simulink model "DAC_SIM_LTE"  (R2013b)
settings: Solver=FixedStepDiscrete  SolverMode=SingleTasking  StartTime=0.0  StopTime=N/Fs  RelTol=1e-3
values from neighbouring files (symbols this model uses):
  Tpass = 1/Fpass    (= 3.25520833333e-08)    [Model.m]
undefined symbols (not defined in the file or in its folder): a1, a2, a3, a4, b1, b2, b3, b4, g1, g2, g3, g4
libraries: xbsIndex_r4 x85, dspmlti4 x3, dspsigops x2, simulink x1
(part 1 of 2)
settings Model: Creator=o_cotte  LastModifiedBy=o_cotte

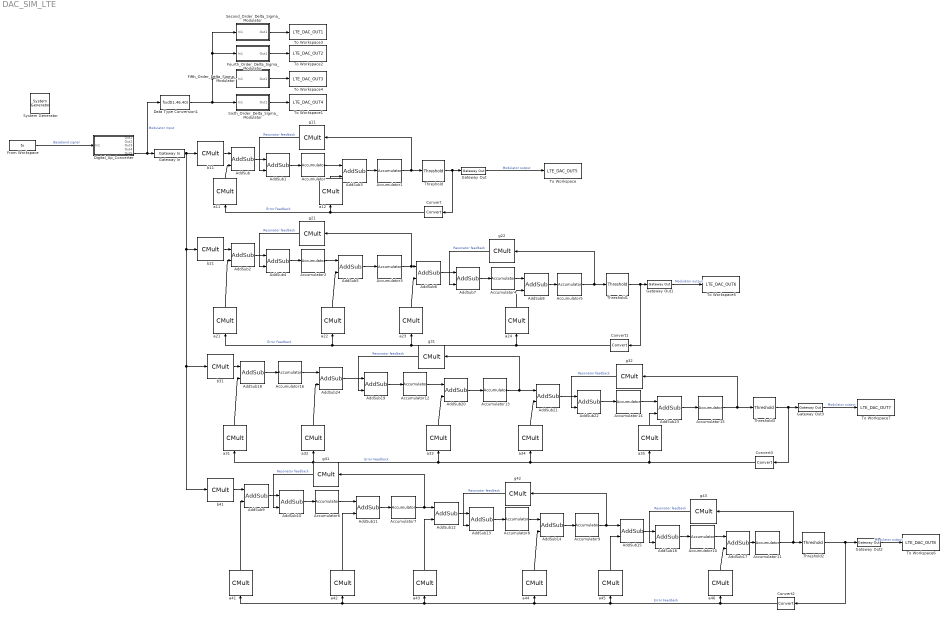
== system DAC_SIM_LTE ==
  " System Generator" : xbsIndex_r4/ System Generator  Tag=genX  xilinxfamily=spartan6  part=xc6slx45  speed=-3  package=csg324  synthesis_tool=XST  clock_wrapper=Clock Enables  directory=./netlist  proj_type=Project Navigator  Synth_file=XST Defaults  Impl_file=ISE Defaults  testbench=off  simulink_period=1/491.52e6  sysclk_period=2.0345052083333335  dcm_input_clock_period=10  incr_netlist=off  trim_vbits=Everywhere in SubSystem  dbl_ovrd=According to Block Masks  core_generation=According to Block Masks  run_coregen=off  deprecated_control=off  eval_field=0  block_type=sysgen
  Accumulator{,1..5,12..16} (11 alike) : xbsIndex_r4/Accumulator  operation=Add  n_bits=46  overflow=Wrap  scale=1  rst=off  infoeditControl=reset for floating point data type must be asserted for a minimum of 2 cycles  hasbypass=off  en=off  latency=0  dbl_ovrd=off  msb_inp=100  msb=100  lsb=-100  use_behavioral_HDL=on  implementation=DSP48  block_type=accum
  Accumulator{6..11} (6 alike) : xbsIndex_r4/Accumulator  operation=Add  n_bits=46  overflow=Wrap  scale=1  rst=off  infoeditControl=reset for floating point data type must be asserted for a minimum of 2 cycles  hasbypass=off  en=off  latency=0  dbl_ovrd=off  msb_inp=100  msb=100  lsb=-100  use_behavioral_HDL=off  implementation=DSP48  block_type=accum
  AddSub{,1..24} (25 alike) : xbsIndex_r4/AddSub  mode=Subtraction  use_carryin=off  use_carryout=off  en=off  latency=0  precision=User Defined  arith_type="Signed  (2's comp)"  n_bits=46  bin_pt=40  quantization=Truncate  overflow=Wrap  dbl_ovrd=off  use_behavioral_HDL=off  hw_selection=DSP48  pipelined=on  block_type=addsub
  Convert{,1..3} (4 alike) : xbsIndex_r4/Convert  gui_display_data_type=Fixed-point  arith_type="Signed  (2's comp)"  n_bits=46  bin_pt=40  float_type=Single  exp_bits=8  fraction_bits=24  quantization=Truncate  overflow=Wrap  en=off  latency=0  dbl_ovrd=off  pipeline=on  block_type=convert
  Data Type Conversion1 : DataTypeConversion  OutDataTypeStr=fixdt(1,46,40)  LockScale=on
  Digital_Up_Converter : Subsystem
  Fifth_Order_Delta_Sigma_Modulator : Subsystem
  Fourth_Order_Delta_Sigma_Modulator : Subsystem
  From Workspace : FromWorkspace  VariableName=tx  SampleTime=Tpass  Interpolate=off  OutputAfterFinalValue=Cyclic repetition
  Gateway In : xbsIndex_r4/Gateway In  gui_display_data_type=Fixed-point  arith_type="Signed  (2's comp)"  n_bits=46  bin_pt=40  preci_type=Single  exp_width=8  frac_width=24  quantization=Truncate  overflow=Saturate  period=1/491.52e6  dbl_ovrd=off  timing_constraint=Data Rate  locs_specified=off  LOCs={}  UseAsADC=off  ADCChannel='1'  inherit_from_input=off  hdl_port=on  block_type=gatewayin
  Gateway Out{,1..3} (4 alike) : xbsIndex_r4/Gateway Out  inherit_from_input=off  hdl_port=on  timing_constraint="Data Rate;  Set 'FAST' Attribute"  locs_specified=off  LOCs={}  UseAsDAC=off  DACChannel='1'  block_type=gatewayout
  Second_Order_Delta_Sigma_Modulator : Subsystem
  Sixth_Order_Delta_Sigma_Modulator : Subsystem
  Threshold{,1..3} (4 alike) : xbsIndex_r4/Threshold  en=off  latency=0  dbl_ovrd=off  block_type=sgn
      settings: infoedit="Presents -1 as output if input is negative; otherwise presents 1.  Output is a two bit signed number."
  To Workspace : ToWorkspace  VariableName=LTE_DAC_OUT5  SampleTime=-1
  To Workspace1 : ToWorkspace  VariableName=LTE_DAC_OUT4  SampleTime=-1
  To Workspace2 : ToWorkspace  VariableName=LTE_DAC_OUT2  SampleTime=-1
  To Workspace3 : ToWorkspace  VariableName=LTE_DAC_OUT1  SampleTime=-1
  To Workspace4 : ToWorkspace  VariableName=LTE_DAC_OUT3  SampleTime=-1
  To Workspace5 : ToWorkspace  VariableName=LTE_DAC_OUT6  SampleTime=-1
  To Workspace6 : ToWorkspace  VariableName=LTE_DAC_OUT8  SampleTime=-1
  To Workspace7 : ToWorkspace  VariableName=LTE_DAC_OUT7  SampleTime=-1
  a11 : xbsIndex_r4/CMult  const=a1(1)  gui_display_data_type=Fixed-point  const_n_bits=46  const_bin_pt=40  float_type=Single  exp_bits=8  fraction_bits=24  en=off  latency=0  precision=User Defined  arith_type="Signed  (2's comp)"  n_bits=46  bin_pt=40  quantization=Truncate  overflow=Wrap  dbl_ovrd=off  use_behavioral_HDL=on  mem_type=Block RAM  pipeline=off  block_type=cmult
  a12 : xbsIndex_r4/CMult  const=a1(2)  gui_display_data_type=Fixed-point  const_n_bits=46  const_bin_pt=40  float_type=Single  exp_bits=8  fraction_bits=24  en=off  latency=0  precision=User Defined  arith_type="Signed  (2's comp)"  n_bits=46  bin_pt=40  quantization=Truncate  overflow=Wrap  dbl_ovrd=off  use_behavioral_HDL=on  mem_type=Block RAM  pipeline=off  block_type=cmult
  a21 : xbsIndex_r4/CMult  const=a2(1)  gui_display_data_type=Fixed-point  const_n_bits=46  const_bin_pt=40  float_type=Single  exp_bits=8  fraction_bits=24  en=off  latency=0  precision=User Defined  arith_type="Signed  (2's comp)"  n_bits=46  bin_pt=40  quantization=Truncate  overflow=Wrap  dbl_ovrd=off  use_behavioral_HDL=on  mem_type=Block RAM  pipeline=off  block_type=cmult
  a22 : xbsIndex_r4/CMult  const=a2(2)  gui_display_data_type=Fixed-point  const_n_bits=46  const_bin_pt=40  float_type=Single  exp_bits=8  fraction_bits=24  en=off  latency=0  precision=User Defined  arith_type="Signed  (2's comp)"  n_bits=46  bin_pt=40  quantization=Truncate  overflow=Wrap  dbl_ovrd=off  use_behavioral_HDL=on  mem_type=Block RAM  pipeline=off  block_type=cmult
  a23 : xbsIndex_r4/CMult  const=a2(3)  gui_display_data_type=Fixed-point  const_n_bits=46  const_bin_pt=40  float_type=Single  exp_bits=8  fraction_bits=24  en=off  latency=0  precision=User Defined  arith_type="Signed  (2's comp)"  n_bits=46  bin_pt=40  quantization=Truncate  overflow=Wrap  dbl_ovrd=off  use_behavioral_HDL=on  mem_type=Block RAM  pipeline=off  block_type=cmult
  a24 : xbsIndex_r4/CMult  const=a2(4)  gui_display_data_type=Fixed-point  const_n_bits=46  const_bin_pt=40  float_type=Single  exp_bits=8  fraction_bits=24  en=off  latency=0  precision=User Defined  arith_type="Signed  (2's comp)"  n_bits=46  bin_pt=40  quantization=Truncate  overflow=Wrap  dbl_ovrd=off  use_behavioral_HDL=on  mem_type=Block RAM  pipeline=off  block_type=cmult
  a31 : xbsIndex_r4/CMult  const=a3(1)  gui_display_data_type=Fixed-point  const_n_bits=46  const_bin_pt=40  float_type=Single  exp_bits=8  fraction_bits=24  en=off  latency=0  precision=User Defined  arith_type="Signed  (2's comp)"  n_bits=46  bin_pt=40  quantization=Truncate  overflow=Wrap  dbl_ovrd=off  use_behavioral_HDL=on  mem_type=Block RAM  pipeline=off  block_type=cmult
  a32 : xbsIndex_r4/CMult  const=a3(2)  gui_display_data_type=Fixed-point  const_n_bits=46  const_bin_pt=40  float_type=Single  exp_bits=8  fraction_bits=24  en=off  latency=0  precision=User Defined  arith_type="Signed  (2's comp)"  n_bits=46  bin_pt=40  quantization=Truncate  overflow=Wrap  dbl_ovrd=off  use_behavioral_HDL=on  mem_type=Block RAM  pipeline=off  block_type=cmult
  a33 : xbsIndex_r4/CMult  const=a3(3)  gui_display_data_type=Fixed-point  const_n_bits=46  const_bin_pt=40  float_type=Single  exp_bits=8  fraction_bits=24  en=off  latency=0  precision=User Defined  arith_type="Signed  (2's comp)"  n_bits=46  bin_pt=40  quantization=Truncate  overflow=Wrap  dbl_ovrd=off  use_behavioral_HDL=on  mem_type=Block RAM  pipeline=off  block_type=cmult
  a34 : xbsIndex_r4/CMult  const=a3(4)  gui_display_data_type=Fixed-point  const_n_bits=46  const_bin_pt=40  float_type=Single  exp_bits=8  fraction_bits=24  en=off  latency=0  precision=User Defined  arith_type="Signed  (2's comp)"  n_bits=46  bin_pt=40  quantization=Truncate  overflow=Wrap  dbl_ovrd=off  use_behavioral_HDL=on  mem_type=Block RAM  pipeline=off  block_type=cmult
  a35 : xbsIndex_r4/CMult  const=a3(5)  gui_display_data_type=Fixed-point  const_n_bits=46  const_bin_pt=40  float_type=Single  exp_bits=8  fraction_bits=24  en=off  latency=0  precision=User Defined  arith_type="Signed  (2's comp)"  n_bits=46  bin_pt=40  quantization=Truncate  overflow=Wrap  dbl_ovrd=off  use_behavioral_HDL=on  mem_type=Block RAM  pipeline=off  block_type=cmult
  a41 : xbsIndex_r4/CMult  const=a4(1)  gui_display_data_type=Fixed-point  const_n_bits=46  const_bin_pt=40  float_type=Single  exp_bits=8  fraction_bits=24  en=off  latency=0  precision=User Defined  arith_type="Signed  (2's comp)"  n_bits=46  bin_pt=40  quantization=Truncate  overflow=Wrap  dbl_ovrd=off  use_behavioral_HDL=on  mem_type=Block RAM  pipeline=off  block_type=cmult
  a42 : xbsIndex_r4/CMult  const=a4(2)  gui_display_data_type=Fixed-point  const_n_bits=46  const_bin_pt=40  float_type=Single  exp_bits=8  fraction_bits=24  en=off  latency=0  precision=User Defined  arith_type="Signed  (2's comp)"  n_bits=46  bin_pt=40  quantization=Truncate  overflow=Wrap  dbl_ovrd=off  use_behavioral_HDL=on  mem_type=Block RAM  pipeline=off  block_type=cmult
  a43 : xbsIndex_r4/CMult  const=a4(3)  gui_display_data_type=Fixed-point  const_n_bits=46  const_bin_pt=40  float_type=Single  exp_bits=8  fraction_bits=24  en=off  latency=0  precision=User Defined  arith_type="Signed  (2's comp)"  n_bits=46  bin_pt=40  quantization=Truncate  overflow=Wrap  dbl_ovrd=off  use_behavioral_HDL=on  mem_type=Block RAM  pipeline=off  block_type=cmult
  a44 : xbsIndex_r4/CMult  const=a4(4)  gui_display_data_type=Fixed-point  const_n_bits=46  const_bin_pt=40  float_type=Single  exp_bits=8  fraction_bits=24  en=off  latency=0  precision=User Defined  arith_type="Signed  (2's comp)"  n_bits=46  bin_pt=40  quantization=Truncate  overflow=Wrap  dbl_ovrd=off  use_behavioral_HDL=on  mem_type=Block RAM  pipeline=off  block_type=cmult
  a45 : xbsIndex_r4/CMult  const=a4(5)  gui_display_data_type=Fixed-point  const_n_bits=46  const_bin_pt=40  float_type=Single  exp_bits=8  fraction_bits=24  en=off  latency=0  precision=User Defined  arith_type="Signed  (2's comp)"  n_bits=46  bin_pt=40  quantization=Truncate  overflow=Wrap  dbl_ovrd=off  use_behavioral_HDL=on  mem_type=Distributed RAM  pipeline=off  block_type=cmult
  a46 : xbsIndex_r4/CMult  const=a4(6)  gui_display_data_type=Fixed-point  const_n_bits=46  const_bin_pt=40  float_type=Single  exp_bits=8  fraction_bits=24  en=off  latency=0  precision=User Defined  arith_type="Signed  (2's comp)"  n_bits=46  bin_pt=40  quantization=Truncate  overflow=Wrap  dbl_ovrd=off  use_behavioral_HDL=on  mem_type=Block RAM  pipeline=off  block_type=cmult
  b11 : xbsIndex_r4/CMult  const=b1(1)  gui_display_data_type=Fixed-point  const_n_bits=46  const_bin_pt=40  float_type=Single  exp_bits=8  fraction_bits=24  en=off  latency=0  precision=User Defined  arith_type="Signed  (2's comp)"  n_bits=46  bin_pt=40  quantization=Truncate  overflow=Wrap  dbl_ovrd=off  use_behavioral_HDL=on  mem_type=Block RAM  pipeline=off  block_type=cmult
  b21 : xbsIndex_r4/CMult  const=b2(1)  gui_display_data_type=Fixed-point  const_n_bits=46  const_bin_pt=40  float_type=Single  exp_bits=8  fraction_bits=24  en=off  latency=0  precision=User Defined  arith_type="Signed  (2's comp)"  n_bits=46  bin_pt=40  quantization=Truncate  overflow=Wrap  dbl_ovrd=off  use_behavioral_HDL=on  mem_type=Block RAM  pipeline=off  block_type=cmult
  b31 : xbsIndex_r4/CMult  const=b3(1)  gui_display_data_type=Fixed-point  const_n_bits=46  const_bin_pt=40  float_type=Single  exp_bits=8  fraction_bits=24  en=off  latency=0  precision=User Defined  arith_type="Signed  (2's comp)"  n_bits=46  bin_pt=40  quantization=Truncate  overflow=Wrap  dbl_ovrd=off  use_behavioral_HDL=on  mem_type=Block RAM  pipeline=off  block_type=cmult
  b41 : xbsIndex_r4/CMult  const=b4(1)  gui_display_data_type=Fixed-point  const_n_bits=46  const_bin_pt=40  float_type=Single  exp_bits=8  fraction_bits=24  en=off  latency=0  precision=User Defined  arith_type="Signed  (2's comp)"  n_bits=46  bin_pt=40  quantization=Truncate  overflow=Wrap  dbl_ovrd=off  use_behavioral_HDL=on  mem_type=Block RAM  pipeline=off  block_type=cmult
  g11 : xbsIndex_r4/CMult  const=g1(1)  gui_display_data_type=Fixed-point  const_n_bits=46  const_bin_pt=40  float_type=Single  exp_bits=8  fraction_bits=24  en=off  latency=0  precision=User Defined  arith_type="Signed  (2's comp)"  n_bits=46  bin_pt=40  quantization=Truncate  overflow=Wrap  dbl_ovrd=off  use_behavioral_HDL=on  mem_type=Block RAM  pipeline=off  block_type=cmult
  g21 : xbsIndex_r4/CMult  const=g2(1)  gui_display_data_type=Fixed-point  const_n_bits=46  const_bin_pt=40  float_type=Single  exp_bits=8  fraction_bits=24  en=off  latency=0  precision=User Defined  arith_type="Signed  (2's comp)"  n_bits=46  bin_pt=40  quantization=Truncate  overflow=Wrap  dbl_ovrd=off  use_behavioral_HDL=on  mem_type=Block RAM  pipeline=off  block_type=cmult
  g22 : xbsIndex_r4/CMult  const=g2(2)  gui_display_data_type=Fixed-point  const_n_bits=46  const_bin_pt=40  float_type=Single  exp_bits=8  fraction_bits=24  en=off  latency=0  precision=User Defined  arith_type="Signed  (2's comp)"  n_bits=46  bin_pt=40  quantization=Truncate  overflow=Wrap  dbl_ovrd=off  use_behavioral_HDL=on  mem_type=Block RAM  pipeline=off  block_type=cmult
  g31 : xbsIndex_r4/CMult  const=g3(1)  gui_display_data_type=Fixed-point  const_n_bits=46  const_bin_pt=40  float_type=Single  exp_bits=8  fraction_bits=24  en=off  latency=0  precision=User Defined  arith_type="Signed  (2's comp)"  n_bits=46  bin_pt=40  quantization=Truncate  overflow=Wrap  dbl_ovrd=off  use_behavioral_HDL=on  mem_type=Block RAM  pipeline=off  block_type=cmult
  g32 : xbsIndex_r4/CMult  const=g3(2)  gui_display_data_type=Fixed-point  const_n_bits=46  const_bin_pt=40  float_type=Single  exp_bits=8  fraction_bits=24  en=off  latency=0  precision=User Defined  arith_type="Signed  (2's comp)"  n_bits=46  bin_pt=40  quantization=Truncate  overflow=Wrap  dbl_ovrd=off  use_behavioral_HDL=on  mem_type=Block RAM  pipeline=off  block_type=cmult
  g41 : xbsIndex_r4/CMult  const=g4(1)  gui_display_data_type=Fixed-point  const_n_bits=46  const_bin_pt=40  float_type=Single  exp_bits=8  fraction_bits=24  en=off  latency=0  precision=User Defined  arith_type="Signed  (2's comp)"  n_bits=46  bin_pt=40  quantization=Truncate  overflow=Wrap  dbl_ovrd=off  use_behavioral_HDL=on  mem_type=Block RAM  pipeline=off  block_type=cmult
  g42 : xbsIndex_r4/CMult  const=g4(2)  gui_display_data_type=Fixed-point  const_n_bits=46  const_bin_pt=40  float_type=Single  exp_bits=8  fraction_bits=24  en=off  latency=0  precision=User Defined  arith_type="Signed  (2's comp)"  n_bits=46  bin_pt=40  quantization=Truncate  overflow=Wrap  dbl_ovrd=off  use_behavioral_HDL=on  mem_type=Block RAM  pipeline=off  block_type=cmult
  g43 : xbsIndex_r4/CMult  const=g4(3)  gui_display_data_type=Fixed-point  const_n_bits=46  const_bin_pt=40  float_type=Single  exp_bits=8  fraction_bits=24  en=off  latency=0  precision=User Defined  arith_type="Signed  (2's comp)"  n_bits=46  bin_pt=40  quantization=Truncate  overflow=Wrap  dbl_ovrd=off  use_behavioral_HDL=on  mem_type=Block RAM  pipeline=off  block_type=cmult
  wires:
  From Workspace/1 -> Digital_Up_Converter/1(In1)  "Baseband signal"
  Digital_Up_Converter/5(Out5) -> Data Type Conversion1/1, Gateway In/1  "Modulator Input"
  g11/1 -> AddSub1/2  "Resonator feedback"
  AddSub/1 -> AddSub1/1
  Gateway Out/1 -> To Workspace/1  "Modulator output"
  Convert/1 -> a12/1, a11/1  "Error Feedback"
  Accumulator/1 -> AddSub3/1
  AddSub1/1 -> Accumulator/1
  a11/1 -> AddSub/2
  a12/1 -> AddSub3/2
  b11/1 -> AddSub/1
  Threshold/1 -> Convert/1, Gateway Out/1
  Accumulator1/1 -> Threshold/1, g11/1
  AddSub3/1 -> Accumulator1/1
  g21/1 -> AddSub4/2  "Resonator feedback"
  AddSub2/1 -> AddSub4/1
  Gateway Out1/1 -> To Workspace5/1  "Modulator output"
  Convert1/1 -> a24/1, a23/1, a22/1, a21/1  "Error Feedback"
  Accumulator2/1 -> AddSub5/1
  AddSub4/1 -> Accumulator2/1
  a21/1 -> AddSub2/2
  a22/1 -> AddSub5/2
  b21/1 -> AddSub2/1
  Threshold1/1 -> Gateway Out1/1, Convert1/1
  AddSub5/1 -> Accumulator3/1
  g22/1 -> AddSub7/2  "Resonator feedback"
  AddSub6/1 -> AddSub7/1
  Accumulator4/1 -> AddSub8/1
  AddSub7/1 -> Accumulator4/1
  a23/1 -> AddSub6/2
  a24/1 -> AddSub8/2
  Accumulator3/1 -> AddSub6/1, g21/1
  Accumulator5/1 -> Threshold1/1, g22/1
  AddSub8/1 -> Accumulator5/1
  g31/1 -> AddSub19/2  "Resonator feedback"
  AddSub18/1 -> Accumulator16/1
  Gateway Out3/1 -> To Workspace7/1  "Modulator output"
  Convert3/1 -> a35/1, a34/1, a32/1, a31/1, a33/1  "Error Feedback"
  Accumulator12/1 -> AddSub20/1
  AddSub19/1 -> Accumulator12/1
  a31/1 -> AddSub18/2
  a33/1 -> AddSub20/2
  b31/1 -> AddSub18/1
  Threshold3/1 -> Gateway Out3/1, Convert3/1
  AddSub20/1 -> Accumulator13/1
  g32/1 -> AddSub22/2  "Resonator feedback"
  AddSub21/1 -> AddSub22/1
  Accumulator14/1 -> AddSub23/1
  AddSub22/1 -> Accumulator14/1
  a34/1 -> AddSub21/2
  a35/1 -> AddSub23/2
  Accumulator13/1 -> AddSub21/1, g31/1
  Accumulator15/1 -> g32/1, Threshold3/1
  AddSub23/1 -> Accumulator15/1
  a32/1 -> AddSub24/2
  Accumulator16/1 -> AddSub24/1
  AddSub24/1 -> AddSub19/1
  g41/1 -> AddSub10/2  "Resonator feedback"
  AddSub9/1 -> AddSub10/1
  Gateway Out2/1 -> To Workspace6/1  "Modulator output"
  Accumulator6/1 -> AddSub11/1
  AddSub10/1 -> Accumulator6/1
  a41/1 -> AddSub9/2
  a42/1 -> AddSub11/2
  b41/1 -> AddSub9/1
  Threshold2/1 -> Convert2/1, Gateway Out2/1
  AddSub11/1 -> Accumulator7/1
  g42/1 -> AddSub13/2  "Resonator feedback"
  AddSub12/1 -> AddSub13/1
  Accumulator8/1 -> AddSub14/1
  AddSub13/1 -> Accumulator8/1
  a43/1 -> AddSub12/2
  a44/1 -> AddSub14/2
  Accumulator7/1 -> AddSub12/1, g41/1
  AddSub14/1 -> Accumulator9/1
  Convert2/1 -> a41/1, a42/1, a43/1, a44/1, a45/1, a46/1  "Error Feedback"
  g43/1 -> AddSub16/2  "Resonator feedback"
  AddSub15/1 -> AddSub16/1
  Accumulator10/1 -> AddSub17/1
  AddSub16/1 -> Accumulator10/1
  a45/1 -> AddSub15/2
  a46/1 -> AddSub17/2
  Accumulator9/1 -> AddSub15/1, g42/1
  Accumulator11/1 -> g43/1, Threshold2/1
  AddSub17/1 -> Accumulator11/1
  Gateway In/1 -> b41/1, b31/1, b21/1, b11/1
  Second_Order_Delta_Sigma_Modulator/1(Out1) -> To Workspace3/1
  Fourth_Order_Delta_Sigma_Modulator/1(Out1) -> To Workspace2/1
  Fifth_Order_Delta_Sigma_Modulator/1(Out1) -> To Workspace4/1
  Sixth_Order_Delta_Sigma_Modulator/1(Out1) -> To Workspace1/1
  Data Type Conversion1/1 -> Second_Order_Delta_Sigma_Modulator/1(In1), Fourth_Order_Delta_Sigma_Modulator/1(In1), Fifth_Order_Delta_Sigma_Modulator/1(In1), Sixth_Order_Delta_Sigma_Modulator/1(In1)

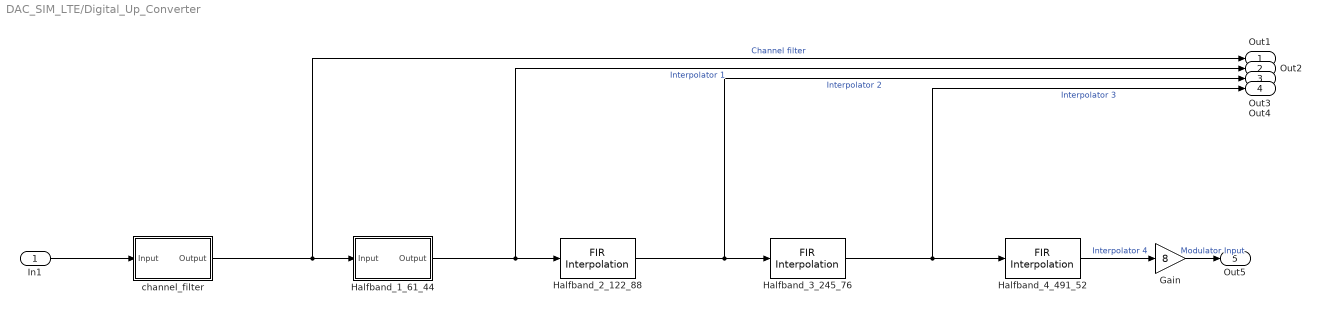
== system DAC_SIM_LTE/Digital_Up_Converter ==
  In1 : Inport
  Gain : Gain  Gain=8
  Halfband_1_61_44 : Subsystem  Tag=FilterWizardSubSystem
      settings: ErrorFcn=dspFilterRealizedInBasicElemsAlgLoopErrFcnCallback
  Halfband_2_122_88 : dspmlti4/FIR Interpolation  Tag=BlockMethodSubSystem  h=[0.0076603622763803236 0 -0.053660411625164647 0 0.29602584582284724 0.5 0.29602584582284724 0 -0.053660411625164647 0 0.0076603622763803236]  L=2  framing=Allow multirate processing  outputBufInitCond=0  firstCoeffDataTypeStr=Inherit: Same word length as input  firstCoeffLastDataTypeStr=Inherit: Same word length as input  firstCoeffMin=[]  firstCoeffMax=[]  outputDataTypeStr=Inherit: Same as accumulator  outputLastDataTypeStr=Inherit: Same as accumulator  outputMin=[]  outputMax=[]  roundingMode=Floor  overflowMode=off  FilterSource=Specify via dialog  FilterObject=Hm_firinterp
  Halfband_3_245_76 : dspmlti4/FIR Interpolation  Tag=BlockMethodSubSystem  h=[-0.032520171835777864 0 0.28248678153183715 0.5 0.28248678153183715 0 -0.032520171835777864]  L=2  framing=Allow multirate processing  outputBufInitCond=0  firstCoeffDataTypeStr=Inherit: Same word length as input  firstCoeffLastDataTypeStr=Inherit: Same word length as input  firstCoeffMin=[]  firstCoeffMax=[]  outputDataTypeStr=Inherit: Same as accumulator  outputLastDataTypeStr=Inherit: Same as accumulator  outputMin=[]  outputMax=[]  roundingMode=Floor  overflowMode=off  FilterSource=Specify via dialog  FilterObject=Hm_firinterp
  Halfband_4_491_52 : dspmlti4/FIR Interpolation  Tag=BlockMethodSubSystem  h=[-0.031562027713033632 0 0.2815599679676668 0.5 0.2815599679676668 0 -0.031562027713033632]  L=2  framing=Allow multirate processing  outputBufInitCond=0  firstCoeffDataTypeStr=Inherit: Same word length as input  firstCoeffLastDataTypeStr=Inherit: Same word length as input  firstCoeffMin=[]  firstCoeffMax=[]  outputDataTypeStr=Inherit: Same as accumulator  outputLastDataTypeStr=Inherit: Same as accumulator  outputMin=[]  outputMax=[]  roundingMode=Floor  overflowMode=off  FilterSource=Specify via dialog  FilterObject=Hm_firinterp
  channel_filter : Subsystem  Tag=FilterWizardSubSystem
      settings: ErrorFcn=dspFilterRealizedInBasicElemsAlgLoopErrFcnCallback
  Out1 : Outport
  Out2 : Outport  Port=2
  Out3 : Outport  Port=3
  Out4 : Outport  Port=4
  Out5 : Outport  Port=5
  wires:
  In1/1 -> channel_filter/1(Input)
  Halfband_1_61_44/1(Output) -> Out2/1, Halfband_2_122_88/1  "Interpolator 1"
  Halfband_2_122_88/1 -> Out3/1, Halfband_3_245_76/1  "Interpolator 2"
  Halfband_4_491_52/1 -> Gain/1  "Interpolator 4"
  Halfband_3_245_76/1 -> Out4/1, Halfband_4_491_52/1  "Interpolator 3"
  Gain/1 -> Out5/1  "Modulator Input"
  channel_filter/1(Output) -> Out1/1, Halfband_1_61_44/1(Input)  "Channel filter"

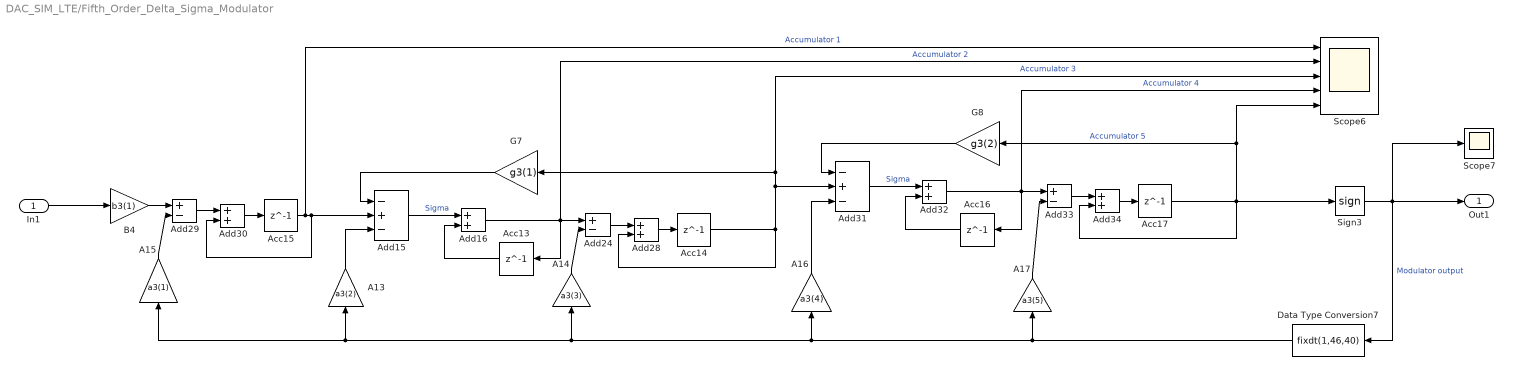
== system DAC_SIM_LTE/Fifth_Order_Delta_Sigma_Modulator ==
  In1 : Inport
  A13 : Gain  Gain=a3(2)  OutDataTypeStr=Inherit: Same as input  ParamDataTypeStr=Inherit: Same as input  LockScale=on
  A14 : Gain  Gain=a3(3)  OutDataTypeStr=Inherit: Same as input  ParamDataTypeStr=Inherit: Same as input  LockScale=on
  A15 : Gain  Gain=a3(1)  OutDataTypeStr=Inherit: Same as input  ParamDataTypeStr=Inherit: Same as input  LockScale=on
  A16 : Gain  Gain=a3(4)  OutDataTypeStr=Inherit: Same as input  ParamDataTypeStr=Inherit: Same as input  LockScale=on
  A17 : Gain  Gain=a3(5)  OutDataTypeStr=Inherit: Same as input  ParamDataTypeStr=Inherit: Same as input  LockScale=on
  Acc{13..17} (5 alike) : Delay  DelayLength=1  InitialCondition=0
  Add15 : Sum  Inputs=-+-  SaturateOnIntegerOverflow=on  InputSameDT=on  OutDataTypeStr=Inherit: Same as first input
  Add{16,28,30,32,34} (5 alike) : Sum  Inputs=2  SaturateOnIntegerOverflow=on  InputSameDT=on  OutDataTypeStr=Inherit: Same as first input
  Add24 : Sum  Inputs=+-  SaturateOnIntegerOverflow=on  InputSameDT=on  OutDataTypeStr=Inherit: Same as first input
  Add29 : Sum  Inputs=+-  SaturateOnIntegerOverflow=on  InputSameDT=on  OutDataTypeStr=Inherit: Same as first input
  Add31 : Sum  Inputs=-+-  SaturateOnIntegerOverflow=on  InputSameDT=on  OutDataTypeStr=Inherit: Same as first input
  Add33 : Sum  Inputs=+-  SaturateOnIntegerOverflow=on  InputSameDT=on  OutDataTypeStr=Inherit: Same as first input
  B4 : Gain  Gain=b3(1)  OutDataTypeStr=Inherit: Same as input  ParamDataTypeStr=Inherit: Same as input  LockScale=on
  Data Type Conversion7 : DataTypeConversion  OutDataTypeStr=fixdt(1,46,40)  LockScale=on
  G7 : Gain  Gain=g3(1)  OutDataTypeStr=Inherit: Same as input  ParamDataTypeStr=Inherit: Same as input  LockScale=on
  G8 : Gain  Gain=g3(2)  OutDataTypeStr=Inherit: Same as input  ParamDataTypeStr=Inherit: Same as input  LockScale=on
  Scope6 : Scope  NumInputPorts=5
  Scope7 : Scope
  Sign3 : Signum
  Out1 : Outport
  wires:
  Acc16/1 -> Add32/2
  A16/1 -> Add31/3
  Add33/1 -> Add34/1
  G8/1 -> Add31/1
  Data Type Conversion7/1 -> A17/1, A14/1, A15/1, A13/1, A16/1
  A17/1 -> Add33/2
  Add31/1 -> Add32/1  "Sigma"
  Acc17/1 -> Sign3/1, Add34/2, Scope6/5, G8/1  "Accumulator 5"
  Add32/1 -> Scope6/4, Add33/1, Acc16/1  "Accumulator 4"
  Add34/1 -> Acc17/1
  Add24/1 -> Add28/1
  Acc13/1 -> Add16/2
  Add29/1 -> Add30/1
  Add30/1 -> Acc15/1
  A13/1 -> Add15/3
  Sign3/1 -> Scope7/1, Out1/1, Data Type Conversion7/1  "Modulator output"
  In1/1 -> B4/1
  Add16/1 -> Scope6/2, Add24/1, Acc13/1  "Accumulator 2"
  A15/1 -> Add29/2
  G7/1 -> Add15/1
  Acc14/1 -> Add31/2, Scope6/3, G7/1, Add28/2  "Accumulator 3"
  Add28/1 -> Acc14/1
  A14/1 -> Add24/2
  Acc15/1 -> Scope6/1, Add15/2, Add30/2  "Accumulator 1"
  Add15/1 -> Add16/1  "Sigma"
  B4/1 -> Add29/1

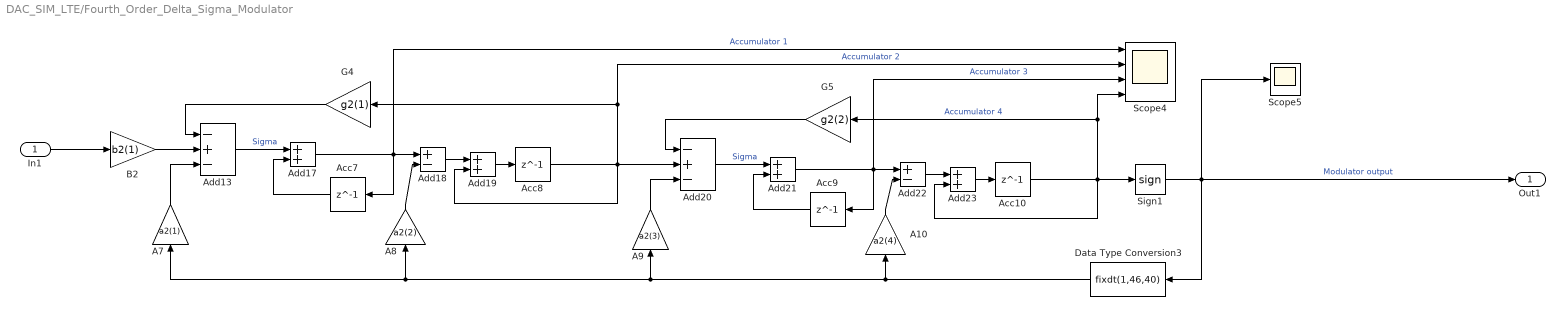
== system DAC_SIM_LTE/Fourth_Order_Delta_Sigma_Modulator ==
  In1 : Inport
  A10 : Gain  Gain=a2(4)  OutDataTypeStr=Inherit: Same as input  ParamDataTypeStr=Inherit: Same as input  LockScale=on
  A7 : Gain  Gain=a2(1)  OutDataTypeStr=Inherit: Same as input  ParamDataTypeStr=Inherit: Same as input  LockScale=on
  A8 : Gain  Gain=a2(2)  OutDataTypeStr=Inherit: Same as input  ParamDataTypeStr=Inherit: Same as input  LockScale=on
  A9 : Gain  Gain=a2(3)  OutDataTypeStr=Inherit: Same as input  ParamDataTypeStr=Inherit: Same as input  LockScale=on
  Acc{7..10} (4 alike) : Delay  DelayLength=1  InitialCondition=0
  Add13 : Sum  Inputs=-+-  SaturateOnIntegerOverflow=on  InputSameDT=on  OutDataTypeStr=Inherit: Same as first input
  Add{17,19,21,23} (4 alike) : Sum  Inputs=2  SaturateOnIntegerOverflow=on  InputSameDT=on  OutDataTypeStr=Inherit: Same as first input
  Add18 : Sum  Inputs=+-  SaturateOnIntegerOverflow=on  InputSameDT=on  OutDataTypeStr=Inherit: Same as first input
  Add20 : Sum  Inputs=-+-  SaturateOnIntegerOverflow=on  InputSameDT=on  OutDataTypeStr=Inherit: Same as first input
  Add22 : Sum  Inputs=+-  SaturateOnIntegerOverflow=on  InputSameDT=on  OutDataTypeStr=Inherit: Same as first input
  B2 : Gain  Gain=b2(1)  OutDataTypeStr=Inherit: Same as input  ParamDataTypeStr=Inherit: Same as input  LockScale=on
  Data Type Conversion3 : DataTypeConversion  OutDataTypeStr=fixdt(1,46,40)  LockScale=on
  G4 : Gain  Gain=g2(1)  OutDataTypeStr=Inherit: Same as input  ParamDataTypeStr=Inherit: Same as input  LockScale=on
  G5 : Gain  Gain=g2(2)  OutDataTypeStr=Inherit: Same as input  ParamDataTypeStr=Inherit: Same as input  LockScale=on
  Scope4 : Scope  NumInputPorts=4
  Scope5 : Scope
  Sign1 : Signum
  Out1 : Outport
  wires:
  Sign1/1 -> Out1/1, Data Type Conversion3/1, Scope5/1  "Modulator output"
  Add13/1 -> Add17/1  "Sigma"
  In1/1 -> B2/1
  Data Type Conversion3/1 -> A10/1, A9/1, A7/1, A8/1
  B2/1 -> Add13/2
  Add17/1 -> Scope4/1, Add18/1, Acc7/1  "Accumulator 1"
  Acc8/1 -> Add20/2, Add19/2, Scope4/2, G4/1  "Accumulator 2"
  A7/1 -> Add13/3
  Acc7/1 -> Add17/2
  Acc10/1 -> Sign1/1, Scope4/4, G5/1, Add23/2  "Accumulator 4"
  Add19/1 -> Acc8/1
  Add18/1 -> Add19/1
  Add22/1 -> Add23/1
  G5/1 -> Add20/1
  Add23/1 -> Acc10/1
  Add21/1 -> Acc9/1, Scope4/3, Add22/1  "Accumulator 3"
  A10/1 -> Add22/2
  A8/1 -> Add18/2
  A9/1 -> Add20/3
  G4/1 -> Add13/1
  Add20/1 -> Add21/1  "Sigma"
  Acc9/1 -> Add21/2

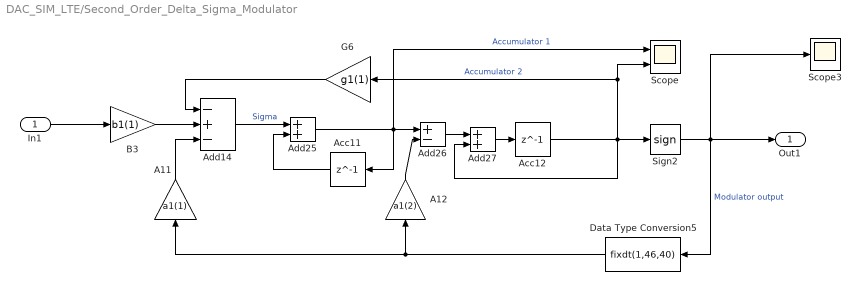
== system DAC_SIM_LTE/Second_Order_Delta_Sigma_Modulator ==
  In1 : Inport
  A11 : Gain  Gain=a1(1)  OutDataTypeStr=Inherit: Same as input  ParamDataTypeStr=Inherit: Same as input  LockScale=on
  A12 : Gain  Gain=a1(2)  OutDataTypeStr=Inherit: Same as input  ParamDataTypeStr=Inherit: Same as input  LockScale=on
  Acc11 : Delay  DelayLength=1  InitialCondition=0
  Acc12 : Delay  DelayLength=1  InitialCondition=0
  Add14 : Sum  Inputs=-+-  SaturateOnIntegerOverflow=on  InputSameDT=on  OutDataTypeStr=Inherit: Same as first input
  Add25 : Sum  Inputs=2  SaturateOnIntegerOverflow=on  InputSameDT=on  OutDataTypeStr=Inherit: Same as first input
  Add26 : Sum  Inputs=+-  SaturateOnIntegerOverflow=on  InputSameDT=on  OutDataTypeStr=Inherit: Same as first input
  Add27 : Sum  Inputs=2  SaturateOnIntegerOverflow=on  InputSameDT=on  OutDataTypeStr=Inherit: Same as first input
  B3 : Gain  Gain=b1(1)  OutDataTypeStr=Inherit: Same as input  ParamDataTypeStr=Inherit: Same as input  LockScale=on
  Data Type Conversion5 : DataTypeConversion  OutDataTypeStr=fixdt(1,46,40)  LockScale=on
  G6 : Gain  Gain=g1(1)  OutDataTypeStr=Inherit: Same as input  ParamDataTypeStr=Inherit: Same as input  LockScale=on
  Scope : Scope  NumInputPorts=2
  Scope3 : Scope
  Sign2 : Signum
  Out1 : Outport
  wires:
  Data Type Conversion5/1 -> A12/1, A11/1
  A11/1 -> Add14/3
  G6/1 -> Add14/1
  B3/1 -> Add14/2
  Acc11/1 -> Add25/2
  Add25/1 -> Scope/1, Add26/1, Acc11/1  "Accumulator 1"
  Acc12/1 -> Sign2/1, Add27/2, Scope/2, G6/1  "Accumulator 2"
  Add27/1 -> Acc12/1
  A12/1 -> Add26/2
  Add26/1 -> Add27/1
  In1/1 -> B3/1
  Add14/1 -> Add25/1  "Sigma"
  Sign2/1 -> Out1/1, Scope3/1, Data Type Conversion5/1  "Modulator output"

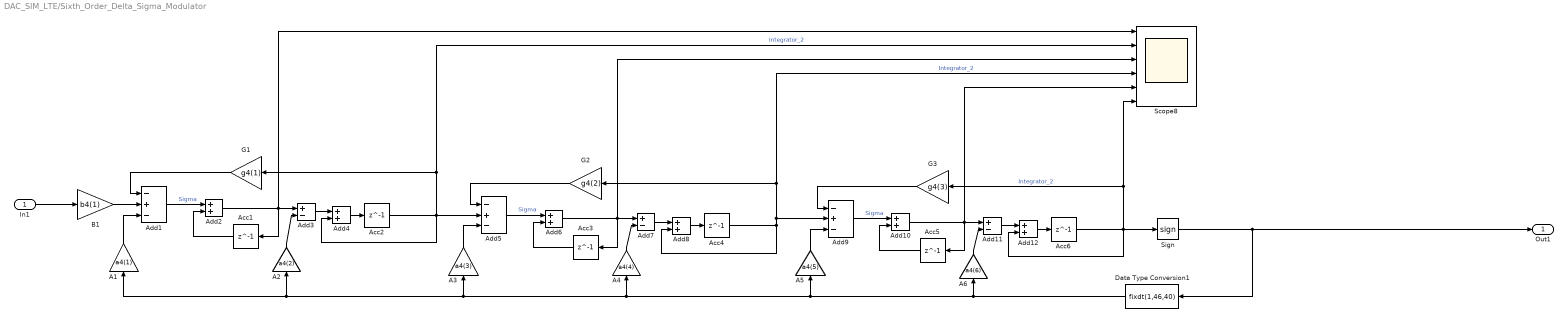
== system DAC_SIM_LTE/Sixth_Order_Delta_Sigma_Modulator ==
  In1 : Inport
  A1 : Gain  Gain=a4(1)  OutDataTypeStr=Inherit: Same as input  ParamDataTypeStr=Inherit: Same as input  LockScale=on
  A2 : Gain  Gain=a4(2)  OutDataTypeStr=Inherit: Same as input  ParamDataTypeStr=Inherit: Same as input  LockScale=on
  A3 : Gain  Gain=a4(3)  OutDataTypeStr=Inherit: Same as input  ParamDataTypeStr=Inherit: Same as input  LockScale=on
  A4 : Gain  Gain=a4(4)  OutDataTypeStr=Inherit: Same as input  ParamDataTypeStr=Inherit: Same as input  LockScale=on
  A5 : Gain  Gain=a4(5)  OutDataTypeStr=Inherit: Same as input  ParamDataTypeStr=Inherit: Same as input  LockScale=on
  A6 : Gain  Gain=a4(6)  OutDataTypeStr=Inherit: Same as input  ParamDataTypeStr=Inherit: Same as input  LockScale=on
  Acc{1..6} (6 alike) : Delay  DelayLength=1  InitialCondition=0
  Add1 : Sum  Inputs=-+-  SaturateOnIntegerOverflow=on  InputSameDT=on  OutDataTypeStr=Inherit: Same as first input
  Add{2,4,6,8,10,12} (6 alike) : Sum  Inputs=2  SaturateOnIntegerOverflow=on  InputSameDT=on  OutDataTypeStr=Inherit: Same as first input
  Add11 : Sum  Inputs=+-  SaturateOnIntegerOverflow=on  InputSameDT=on  OutDataTypeStr=Inherit: Same as first input
  Add3 : Sum  Inputs=+-  SaturateOnIntegerOverflow=on  InputSameDT=on  OutDataTypeStr=Inherit: Same as first input
  Add5 : Sum  Inputs=-+-  SaturateOnIntegerOverflow=on  InputSameDT=on  OutDataTypeStr=Inherit: Same as first input
  Add7 : Sum  Inputs=+-  SaturateOnIntegerOverflow=on  InputSameDT=on  OutDataTypeStr=Inherit: Same as first input
  Add9 : Sum  Inputs=-+-  SaturateOnIntegerOverflow=on  InputSameDT=on  OutDataTypeStr=Inherit: Same as first input
  B1 : Gain  Gain=b4(1)  OutDataTypeStr=Inherit: Same as input  ParamDataTypeStr=Inherit: Same as input  LockScale=on
  Data Type Conversion1 : DataTypeConversion  OutDataTypeStr=fixdt(1,46,40)  LockScale=on
  G1 : Gain  Gain=g4(1)  OutDataTypeStr=Inherit: Same as input  ParamDataTypeStr=Inherit: Same as input  LockScale=on
  G2 : Gain  Gain=g4(2)  OutDataTypeStr=Inherit: Same as input  ParamDataTypeStr=Inherit: Same as input  LockScale=on
  G3 : Gain  Gain=g4(3)  OutDataTypeStr=Inherit: Same as input  ParamDataTypeStr=Inherit: Same as input  LockScale=on
  Scope8 : Scope  NumInputPorts=6
  Sign : Signum
  Out1 : Outport
  wires:
  Add1/1 -> Add2/1  "Sigma"
  Sign/1 -> Out1/1, Data Type Conversion1/1
  In1/1 -> B1/1
  Data Type Conversion1/1 -> A6/1, A4/1, A1/1, A2/1, A3/1, A5/1
  B1/1 -> Add1/2
  A1/1 -> Add1/3
  Acc1/1 -> Add2/2
  Add2/1 -> Scope8/1, Add3/1, Acc1/1
  Add4/1 -> Acc2/1
  G1/1 -> Add1/1
  Acc2/1 -> Add5/2, Add4/2, Scope8/2, G1/1  "Integrator_2"
  Add3/1 -> Add4/1
  A2/1 -> Add3/2
  Add5/1 -> Add6/1  "Sigma"
  A3/1 -> Add5/3
  Add11/1 -> Add12/1
  G3/1 -> Add9/1
  Add6/1 -> Scope8/3, Add7/1, Acc3/1
  A6/1 -> Add11/2
  Acc3/1 -> Add6/2
  Acc4/1 -> Add9/2, Scope8/4, G2/1, Add8/2  "Integrator_2"
  Add9/1 -> Add10/1  "Sigma"
  Add7/1 -> Add8/1
  A5/1 -> Add9/3
  Add10/1 -> Scope8/5, Add11/1, Acc5/1
  Add12/1 -> Acc6/1
  Acc6/1 -> Sign/1, Add12/2, Scope8/6, G3/1  "Integrator_2"
  Acc5/1 -> Add10/2
  Add8/1 -> Acc4/1
  G2/1 -> Add5/1
  A4/1 -> Add7/2

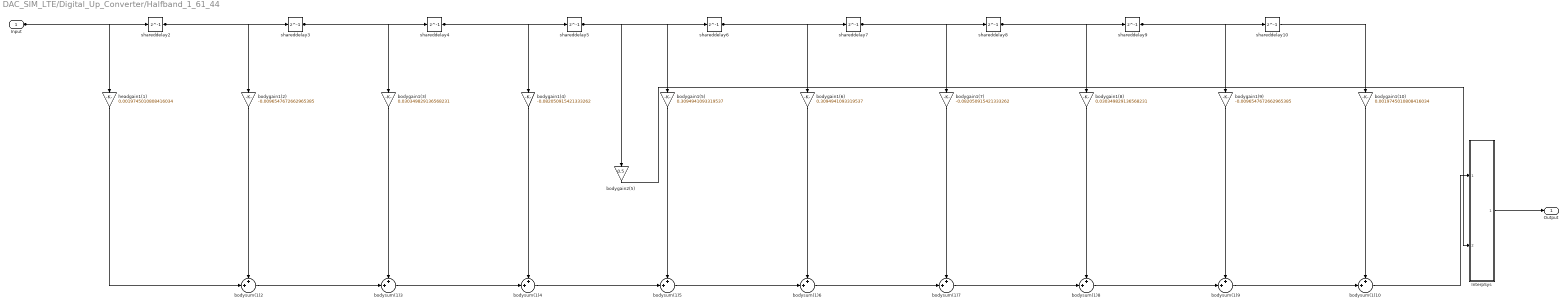
== system DAC_SIM_LTE/Digital_Up_Converter/Halfband_1_61_44 ==
  Input : Inport
  InterpSys : Subsystem  Tag=FilterWizardInterpolatorCommutator
  bodygain1(10) : Gain  Gain=0.0019745010808416034  ParamDataTypeStr=double  RndMeth=Nearest  SaturateOnIntegerOverflow=on  OutDataTypeStr=Inherit: Same as input
  bodygain1(2) : Gain  Gain=-0.0096547672662965385  ParamDataTypeStr=double  RndMeth=Nearest  SaturateOnIntegerOverflow=on  OutDataTypeStr=Inherit: Same as input
  bodygain1(3) : Gain  Gain=0.030349829136568231  ParamDataTypeStr=double  RndMeth=Nearest  SaturateOnIntegerOverflow=on  OutDataTypeStr=Inherit: Same as input
  bodygain1(4) : Gain  Gain=-0.082050915421333262  ParamDataTypeStr=double  RndMeth=Nearest  SaturateOnIntegerOverflow=on  OutDataTypeStr=Inherit: Same as input
  bodygain1(5) : Gain  Gain=0.3094941093319537  ParamDataTypeStr=double  RndMeth=Nearest  SaturateOnIntegerOverflow=on  OutDataTypeStr=Inherit: Same as input
  bodygain1(6) : Gain  Gain=0.3094941093319537  ParamDataTypeStr=double  RndMeth=Nearest  SaturateOnIntegerOverflow=on  OutDataTypeStr=Inherit: Same as input
  bodygain1(7) : Gain  Gain=-0.082050915421333262  ParamDataTypeStr=double  RndMeth=Nearest  SaturateOnIntegerOverflow=on  OutDataTypeStr=Inherit: Same as input
  bodygain1(8) : Gain  Gain=0.030349829136568231  ParamDataTypeStr=double  RndMeth=Nearest  SaturateOnIntegerOverflow=on  OutDataTypeStr=Inherit: Same as input
  bodygain1(9) : Gain  Gain=-0.0096547672662965385  ParamDataTypeStr=double  RndMeth=Nearest  SaturateOnIntegerOverflow=on  OutDataTypeStr=Inherit: Same as input
  bodygain2(5) : Gain  Gain=0.5  ParamDataTypeStr=double  RndMeth=Nearest  SaturateOnIntegerOverflow=on  OutDataTypeStr=Inherit: Same as input
  bodysum(1){2..10} (9 alike) : Sum  Inputs=++|  RndMeth=Nearest  SaturateOnIntegerOverflow=on  OutDataTypeStr=Inherit: Same as first input
  headgain1(1) : Gain  Gain=0.0019745010808416034  ParamDataTypeStr=double  RndMeth=Nearest  SaturateOnIntegerOverflow=on  OutDataTypeStr=Inherit: Same as input
  shareddelay{2..10} (9 alike) : Delay  DelayLength=1  InitialCondition=0
  Output : Outport
  wires:
  headgain1(1)/1 -> bodysum(1)2/2
  Input/1 -> headgain1(1)/1, shareddelay2/1
  bodygain1(2)/1 -> bodysum(1)2/1
  bodysum(1)2/1 -> bodysum(1)3/2
  shareddelay2/1 -> bodygain1(2)/1, shareddelay3/1
  bodygain1(3)/1 -> bodysum(1)3/1
  bodysum(1)3/1 -> bodysum(1)4/2
  shareddelay3/1 -> bodygain1(3)/1, shareddelay4/1
  bodygain1(4)/1 -> bodysum(1)4/1
  bodysum(1)4/1 -> bodysum(1)5/2
  shareddelay4/1 -> bodygain1(4)/1, shareddelay5/1
  bodygain1(5)/1 -> bodysum(1)5/1
  bodygain2(5)/1 -> InterpSys/2(input2)
  bodysum(1)5/1 -> bodysum(1)6/2
  shareddelay5/1 -> bodygain1(5)/1, bodygain2(5)/1, shareddelay6/1
  bodygain1(6)/1 -> bodysum(1)6/1
  bodysum(1)6/1 -> bodysum(1)7/2
  shareddelay6/1 -> bodygain1(6)/1, shareddelay7/1
  bodygain1(7)/1 -> bodysum(1)7/1
  bodysum(1)7/1 -> bodysum(1)8/2
  shareddelay7/1 -> bodygain1(7)/1, shareddelay8/1
  bodygain1(8)/1 -> bodysum(1)8/1
  bodysum(1)8/1 -> bodysum(1)9/2
  shareddelay8/1 -> bodygain1(8)/1, shareddelay9/1
  bodygain1(9)/1 -> bodysum(1)9/1
  bodysum(1)9/1 -> bodysum(1)10/2
  shareddelay9/1 -> bodygain1(9)/1, shareddelay10/1
  bodygain1(10)/1 -> bodysum(1)10/1
  bodysum(1)10/1 -> InterpSys/1(input1)
  shareddelay10/1 -> bodygain1(10)/1
  InterpSys/1(output) -> Output/1
